simulink model "blockKicker_tIB"  (R2014b)
settings: Solver=FixedStepDiscrete  StartTime=0.0  StopTime=10.0  RelTol=1e-3
libraries: c2833xlib x4, simulink x3, c280xlib x2
settings Model: Creator=Michael  LastModifiedBy=Michael
settings DataIOCC: SaveOutput=off  SaveTime=off
settings OptimizationCC: OptimizeModelRefInitCode=on  LifeSpan=1
settings HardwareCC: ProdBitPerChar=16  ProdBitPerInt=16  ProdBitPerPointer=16  ProdLargestAtomicInteger=Integer  ProdIntDivRoundTo=Zero  ProdEndianess=LittleEndian  ProdWordSize=16  ProdHWDeviceType=Texas Instruments->C2000
settings RTWCC: SystemTargetFile=idelink_ert.tlc  GenerateMakefile=off  TemplateMakefile=none  Description=IDE Link ERT  ProcessScript=idelink_ert_make_rtw_hook  Toolchain=Texas Instruments Code Composer Studio v5 (C2000)
settings CodeAppCC: IgnoreCustomStorageClasses=off
settings TargetHardwareResources: Description=Target Hardware Resources Component

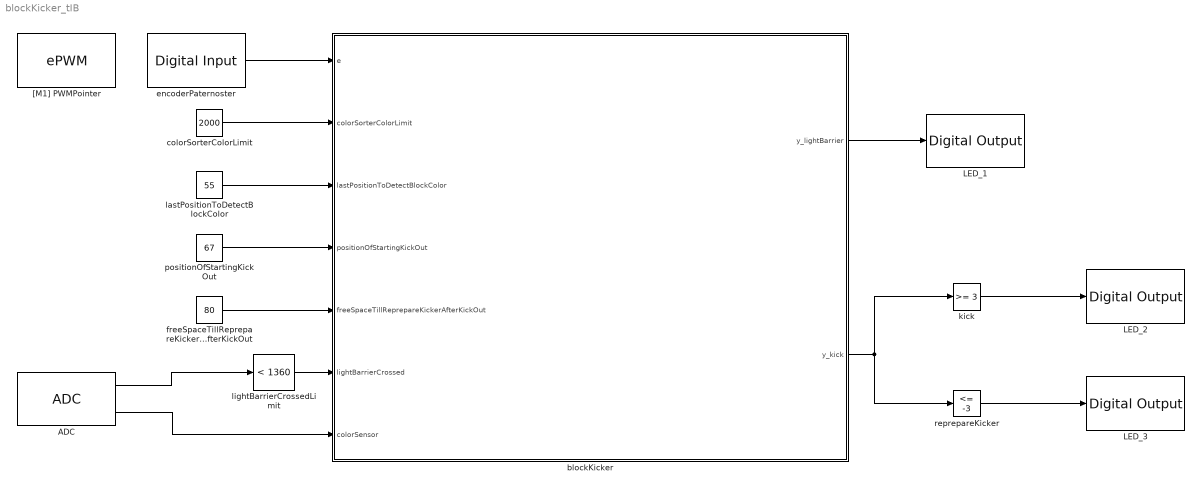
== system blockKicker_tIB ==
  ADC : c280xlib/ADC  useModule=A  useMode=Sequential  sourceSOC=Software  sourceSOC1=Software  sourceSOC2=ePWMxB  xint2_ADCSOC=31  Ts=0.001  dType=uint16  postInterrupt=off  numConversionsSingle=2  numConversionsDouble=1  conv0=ADCINA0  conv1=ADCINA1  conv2=ADCINA2  conv3=ADCINA3  conv4=ADCINA4  conv5=ADCINA5  conv6=ADCINA6  conv7=ADCINA7  conv8=ADCINB0  conv9=ADCINB1  conv10=ADCINB2  conv11=ADCINB3  conv12=ADCINB4  conv13=ADCINB5  conv14=ADCINB6  conv15=ADCINB7  convAB0=ADCINA0 and ADCINB0  convAB1=ADCINA1 and ADCINB1  convAB2=ADCINA2 and ADCINB2  convAB3=ADCINA3 and ADCINB3  convAB4=ADCINA4 and ADCINB4  convAB5=ADCINA5 and ADCINB5  convAB6=ADCINA6 and ADCINB6  convAB7=ADCINA7 and ADCINB7  convA0=ADCINA0  convA1=ADCINA1  convA2=ADCINA2  convA3=ADCINA3  convA4=ADCINA4  convA5=ADCINA5  convA6=ADCINA6  convA7=ADCINA7  convB0=ADCINB0  convB1=ADCINB1  convB2=ADCINB2  convB3=ADCINB3  convB4=ADCINB4  convB5=ADCINB5  convB6=ADCINB6  convB7=ADCINB7  c28xmultiPort=on  endma=off  chdma=1
  LED_1 : c2833xlib/Digital Output  GPIO_Number=GPIO56~GPIO63  GPIO_Bit0=off  GPIO_BIT0_Toggle=off  GPIO_Bit1=off  GPIO_BIT1_Toggle=off  GPIO_Bit2=on  GPIO_BIT2_Toggle=off  GPIO_Bit3=off  GPIO_BIT3_Toggle=off  GPIO_Bit4=off  GPIO_BIT4_Toggle=off  GPIO_Bit5=off  GPIO_BIT5_Toggle=off  GPIO_Bit6=off  GPIO_BIT6_Toggle=off  GPIO_Bit7=off  GPIO_BIT7_Toggle=off
  LED_2 : c2833xlib/Digital Output  GPIO_Number=GPIO56~GPIO63  GPIO_Bit0=off  GPIO_BIT0_Toggle=off  GPIO_Bit1=off  GPIO_BIT1_Toggle=off  GPIO_Bit2=off  GPIO_BIT2_Toggle=off  GPIO_Bit3=on  GPIO_BIT3_Toggle=off  GPIO_Bit4=off  GPIO_BIT4_Toggle=off  GPIO_Bit5=off  GPIO_BIT5_Toggle=off  GPIO_Bit6=off  GPIO_BIT6_Toggle=off  GPIO_Bit7=off  GPIO_BIT7_Toggle=off
  LED_3 : c2833xlib/Digital Output  GPIO_Number=GPIO56~GPIO63  GPIO_Bit0=off  GPIO_BIT0_Toggle=off  GPIO_Bit1=off  GPIO_BIT1_Toggle=off  GPIO_Bit2=off  GPIO_BIT2_Toggle=off  GPIO_Bit3=off  GPIO_BIT3_Toggle=off  GPIO_Bit4=on  GPIO_BIT4_Toggle=off  GPIO_Bit5=off  GPIO_BIT5_Toggle=off  GPIO_Bit6=off  GPIO_BIT6_Toggle=off  GPIO_Bit7=off  GPIO_BIT7_Toggle=off
  "[M1] PWMPointer" : c280xlib/ePWM  checkMode=off  useModule=ePWM2  periodUnits=Clock cycles  timerSource=Specify via dialog  timerPeriod_clk=64000  timerPeriod_sec=0.0001  tbshadow=Counter equals to zero  countingMode=Up  phaseActiveEnable=Disable  phaseDirection=Count down after sync  phaseActive=0  synchronizationEnable=off  synchronizationOption=Disable  clockPrescale=1  HSclockPrescale=1  ePWMxAStatus=off  CMPAUnits=Clock cycles  CMPASource=Specify via dialog  CMPAValue_per=50  CMPAValue_clk=32000  enCMPAshadow=Counter equals to zero  ePWMxAactionLogic1=Do nothing  ePWMxAactionLogic2=Clear  ePWMxAactionLogic3=Set  ePWMxAactionLogic4=Do nothing  ePWMxAactionLogic5=Do nothing  ePWMxAactionLogic6=Do nothing  ePWMxALoadMode=Load on counter equals to zero (CTR=Zero)  ePWMxACSFenable=off  ePWMxACSFvalue=Forcing disable  ePWMxASFreload=Zero  enHRPWM=off  HRPWM_LoadMode=Counter equals to zero (CTR=ZERO)  HRPWM_CTLMode=Phase control mode  HRPWM_EDGMode=Both edge  enSFO=on  ePWMxBStatus=on  CMPBUnits=Percentages  CMPBSource=Specify via dialog  CMPBValue_per=80  CMPBValue_clk=32000  enCMPBshadow=Counter equals to zero  ePWMxBactionLogic1=Do nothing  ePWMxBactionLogic2=Set  ePWMxBactionLogic3=Do nothing  ePWMxBactionLogic4=Do nothing  ePWMxBactionLogic5=Clear  ePWMxBactionLogic6=Do nothing  ePWMxBLoadMode=Load on counter equals to zero (CTR=Zero)  ePWMxBCSFenable=off  ePWMxBCSFvalue=Forcing disable  ePWMxBSFreload=Zero  enableDBePWMxA=off  enableDBePWMxB=off  DBpolarity=Active high (AH)  DBedgeDelay=Positive  DBSource_ePWMxA=ePWMxA  DBSource_ePWMxB=ePWMxA  DBperiodSource=Specify via dialog  REDperiod=0  FEDperiod=0  adcstartModuleA=off  adcrequestEventA=First event  adcstartEventA=Counter equals to zero (CTR=Zero)  adcstartModuleB=off  adcrequestEventB=First event  adcstartEventB=Counter equals to zero (CTR=Zero)  intEn=off  intPrd=First event  intSel=Counter equals to zero (CTR=Zero)  chopperEnable=off  chopperFrequency=1  chopperFirstwidth=1  chopperDuty=12.5%  tripZonesource=Specify via dialog  tzselOSHT1=off  tzselOSHT2=off  tzselOSHT3=off  tzselOSHT4=off  tzselOSHT5=off  tzselOSHT6=off  tzselCBC1=off  tzselCBC2=off  tzselCBC3=off  tzselCBC4=off  tzselCBC5=off  tzselCBC6=off  enTzOstIntr=off  enTzCbcIntr=off  ePWMxAforced=No action  ePWMxBforced=No action  timerPeriod=-1  ePWMxAValue=0  ePWMxBValue=0  tripZoneoption=One-shot trip (OSHT)
  blockKicker : Stateflow chart  TreatAsAtomicUnit=on
  colorSorterColorLimit : Constant  Value=2000  OutMin=0  OutMax=4095  OutDataTypeStr=uint16
  encoderPaternoster : c2833xlib/Digital Input  GPIO_Number=GPIO24~GPIO31  GPIO_Bit0=off  GPIO_Bit1=on  GPIO_Bit2=off  GPIO_Bit3=off  GPIO_Bit4=off  GPIO_Bit5=off  GPIO_Bit6=off  GPIO_Bit7=off  sampleTime=0.001  dataType=auto  GPIO_Bit0_Qualification=Sync to SYSCLKOUT  GPIO_Bit1_Qualification=Sync to SYSCLKOUT  GPIO_Bit2_Qualification=Sync to SYSCLKOUT  GPIO_Bit3_Qualification=Sync to SYSCLKOUT  GPIO_Bit4_Qualification=Sync to SYSCLKOUT  GPIO_Bit5_Qualification=Sync to SYSCLKOUT  GPIO_Bit6_Qualification=Sync to SYSCLKOUT  GPIO_Bit7_Qualification=Sync to SYSCLKOUT  Qualification_Period=-1
  freeSpaceTillReprepareKickerAfterKickOut : Constant  Value=80  OutDataTypeStr=uint32
  kick : simulink/Logic and Bit Operations/Compare To Constant  relop=>=  const=3  OutDataTypeStr=boolean
  lastPositionToDetectBlockColor : Constant  Value=55  OutDataTypeStr=uint32
  lightBarrierCrossedLimit : simulink/Logic and Bit Operations/Compare To Constant  relop=<  const=1360  OutDataTypeStr=boolean
  positionOfStartingKickOut : Constant  Value=67  OutDataTypeStr=uint32
  reprepareKicker : simulink/Logic and Bit Operations/Compare To Constant  relop=<=  const=-3  OutDataTypeStr=boolean
  wires:
  encoderPaternoster/1 -> blockKicker/1(e)
  ADC/1 -> lightBarrierCrossedLimit/1
  lightBarrierCrossedLimit/1 -> blockKicker/6(lightBarrierCrossed)
  blockKicker/1(y_lightBarrier) -> LED_1/1
  freeSpaceTillReprepareKickerAfterKickOut/1 -> blockKicker/5(freeSpaceTillReprepareKickerAfterKickOut)
  positionOfStartingKickOut/1 -> blockKicker/4(positionOfStartingKickOut)
  lastPositionToDetectBlockColor/1 -> blockKicker/3(lastPositionToDetectBlockColor)
  colorSorterColorLimit/1 -> blockKicker/2(colorSorterColorLimit)
  blockKicker/2(y_kick) -> reprepareKicker/1, kick/1
  kick/1 -> LED_2/1
  reprepareKicker/1 -> LED_3/1
  ADC/2 -> blockKicker/7(colorSensor)

== stateflow chart blockKicker_tIB/blockKicker ==
  state lightBarrier_controller [parallel]
    settings: executionOrder=3
    state idle
      entry: y_lightBarrier = false;
    state lightBarrierCrossed
      entry: send(counterFromLightBarrierCrossed.RESET);
      send(color_controller.NEXTBLOCK);
      y_lightBarrier = true;
    (default) -> lightBarrier_controller.idle : /{kicker_controller.enqueuedBlocksToKick =uint8( 0)}
    lightBarrier_controller.idle -> lightBarrierCrossed : [lightBarrierCrossed >= 1]
    lightBarrierCrossed -> lightBarrier_controller.idle : [lightBarrierCrossed <1]
  state counterFromLightBarrierCrossed [parallel]
    settings: executionOrder=1
    state start
      entry: count= uint32(0);
    state highLevel
    state lowLevel
      entry: count = count + 1;
    counterFromLightBarrierCrossed.lowLevel -> counterFromLightBarrierCrossed.highLevel : [e>0]
    (default) -> counterFromLightBarrierCrossed.start
    counterFromLightBarrierCrossed.start -> counterFromLightBarrierCrossed.lowLevel : [e>0]
    counterFromLightBarrierCrossed.highLevel -> counterFromLightBarrierCrossed.lowLevel : [e==0]
    counterFromLightBarrierCrossed -> counterFromLightBarrierCrossed.start : RESET
  state counterFromKick [parallel]
    settings: executionOrder=2
    state start
      entry: count= uint32(0);
    state highLevel
    state lowLevel
      entry: count = count + 1;
    counterFromKick.lowLevel -> counterFromKick.highLevel : [e>0]
    (default) -> counterFromKick.start
    counterFromKick.start -> counterFromKick.lowLevel : [e>0]
    counterFromKick.highLevel -> counterFromKick.lowLevel : [e==0]
    counterFromKick -> counterFromKick.start : RESET
  state kicker_controller [parallel]
    settings: executionOrder=5
    state kick
      entry: send(counterFromKick.RESET);
      enqueuedBlocksToKick = enqueuedBlocksToKick -1;
      y_kick = int16(5);
    state idle
      entry: y_kick = int16(0);
    state reprepareKicker
      entry: y_kick = int16(-5);
    (default) -> kicker_controller.idle
    kicker_controller.idle -> kick : [[counterFromLightBarrierCrossed.count >= positionOfStartingKickOut] && [enqueuedBlocksToKick > 0]]
    reprepareKicker -> kicker_controller.idle
    kick -> reprepareKicker : [counterFromKick.count >= freeSpaceTillReprepareKickerAfterKickOut]
  state color_controller [parallel]
    settings: executionOrder=4
    state blockToKick
      entry: kicker_controller.enqueuedBlocksToKick = kicker_controller.enqueuedBlocksToKick + 1;
    state blockNotToKick
    state waitingForBlockToPassColorSensor
    (default) -> blockNotToKick
    waitingForBlockToPassColorSensor -> (junction 89) [order 1] : [counterFromLightBarrierCrossed.count >= lastPositionToDetectBlockColor]
    (junction 89) -> blockToKick [order 1] : [shouldBeKicked == true]
    blockNotToKick -> waitingForBlockToPassColorSensor : NEXTBLOCK /{shouldBeKicked = true}
    (junction 89) -> (junction 91) [order 2] : [shouldBeKicked == false]
    waitingForBlockToPassColorSensor -> waitingForBlockToPassColorSensor [order 2] : [colorSensor <= colorSorterColorLimit] {shouldBeKicked = false}
    (junction 91) -> blockNotToKick
    blockToKick -> (junction 91)
  data: count local uint32; count local uint32; enqueuedBlocksToKick local uint8 [0..2]; shouldBeKicked local boolean; e input; y_lightBarrier output boolean; y_kick output int16; colorSorterColorLimit input uint16 [0..4095]; lastPositionToDetectBlockColor input uint32; positionOfStartingKickOut input uint32; freeSpaceTillReprepareKickerAfterKickOut input uint32; lightBarrierCrossed input; colorSensor input uint16 [0..4095]
  data lastPositionToDetectBlockColor settings: description=length from light barrier to last possible position for color detection of blocks in tics from encoder
  data positionOfStartingKickOut settings: description=length from light barrier to position where kicker starts off kicking out blocks in tics from encoder
  data freeSpaceTillReprepareKickerAfterKickOut settings: description=space to wait after the kick out of a block till kicker reprepares (crosses the drive lane again) in tics from encoder
  events: RESET local FUNCTION_CALL_EVENT; RESET local FUNCTION_CALL_EVENT; NEXTBLOCK local FUNCTION_CALL_EVENT
